simulink library "lib_orbittrance"  (Simulink 7.7)
settings: Solver=ode45  StartTime=0.0  StopTime=10.0  RelTol=1e-3
undefined symbols (not defined in the file): Earth, earth_radius, WGS84
libraries: aerolibutil x7, lib_util x4, vrlib x4, lib_orbittrance x4, lib_astrodynamics x3, aerolibtransform2 x2, lib_env x1
settings Model: Creator=miyata  LastModifiedBy=yamaurashusaku

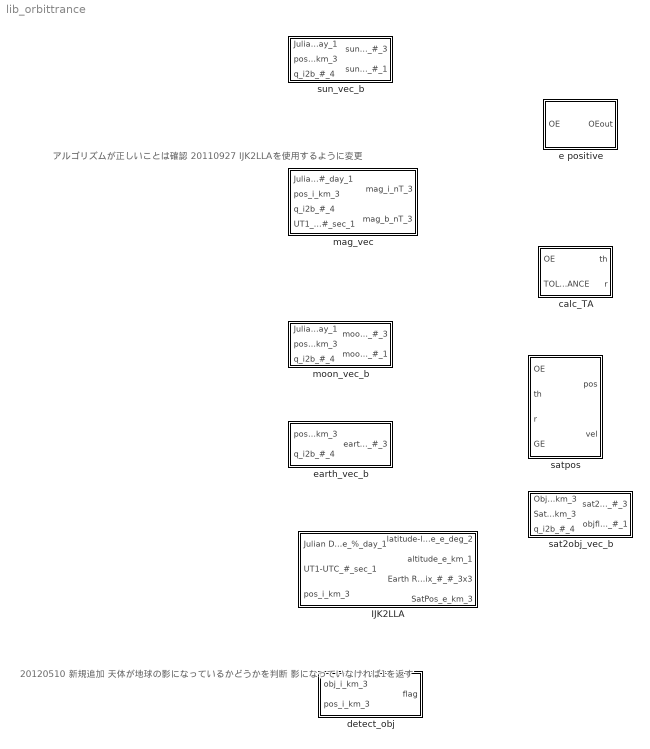
== system lib_orbittrance ==
  note: アルゴリズムが正しいことは確認
      | 20110927 IJK2LLAを使用するように変更
  note: 20120510 新規追加
      | 天体が地球の影になっているかどうかを判断
      | 影になっていなければ1を返す
  IJK2LLA : Subsystem
  calc_TA : Stateflow chart  TreatAsAtomicUnit=on
  detect_obj : Subsystem
  e positive : Stateflow chart  TreatAsAtomicUnit=on
  earth_vec_b : Subsystem
  mag_vec : Subsystem
  moon_vec_b : Subsystem
  sat2obj_vec_b : Subsystem
  satpos : Stateflow chart  TreatAsAtomicUnit=on
  sun_vec_b : Subsystem

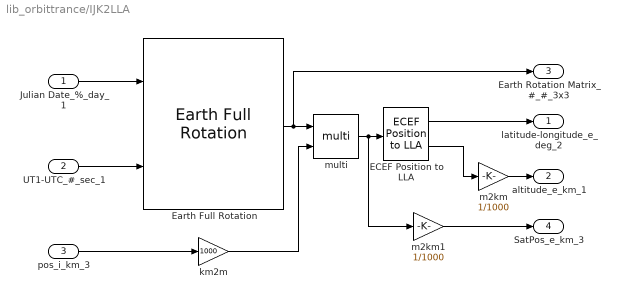
== system lib_orbittrance/IJK2LLA ==
  Julian Date_%_day_1 : Inport
  UT1-UTC_#_sec_1 : Inport  Port=2
  pos_i_km_3 : Inport  Port=3
  ECEF Position to LLA : aerolibtransform2/ECEF Position to LLA  units=Metric (MKS)  ptype=Earth (WGS84)  F=1/298.257223563  R=6378137
  Earth Full Rotation : lib_astrodynamics/Earth Full Rotation
  km2m : Gain  Gain=1000
  m2km : Gain  Gain=1/1000
  m2km1 : Gain  Gain=1/1000
  multi : lib_util/multi
  latitude-longitude_e_deg_2 : Outport
  altitude_e_km_1 : Outport  Port=2
  Earth Rotation Matrix_#_#_3x3 : Outport  Port=3
  SatPos_e_km_3 : Outport  Port=4
  wires:
  Julian Date_%_day_1/1 -> Earth Full Rotation/1
  UT1-UTC_#_sec_1/1 -> Earth Full Rotation/2
  pos_i_km_3/1 -> km2m/1
  Earth Full Rotation/1 -> multi/1, Earth Rotation Matrix_#_#_3x3/1
  km2m/1 -> multi/2
  multi/1 -> ECEF Position to LLA/1, m2km1/1
  ECEF Position to LLA/1 -> latitude-longitude_e_deg_2/1
  ECEF Position to LLA/2 -> m2km/1
  m2km/1 -> altitude_e_km_1/1
  m2km1/1 -> SatPos_e_km_3/1

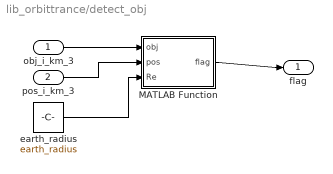
== system lib_orbittrance/detect_obj ==
  obj_i_km_3 : Inport
  pos_i_km_3 : Inport  Port=2
  MATLAB Function : Stateflow chart  TreatAsAtomicUnit=on
  earth_radius : Constant  Value=earth_radius
  flag : Outport
  wires:
  MATLAB Function/1(flag) -> flag/1
  obj_i_km_3/1 -> MATLAB Function/1(obj)
  pos_i_km_3/1 -> MATLAB Function/2(pos)
  earth_radius/1 -> MATLAB Function/3(Re)

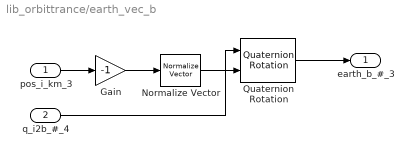
== system lib_orbittrance/earth_vec_b ==
  pos_i_km_3 : Inport
  q_i2b_#_4 : Inport  Port=2
  Gain : Gain  Gain=-1
  Normalize Vector : vrlib/Utilities/Normalize Vector  maxzero=0
  Quaternion Rotation : aerolibutil/Quaternion Rotation
  earth_b_#_3 : Outport
  wires:
  Normalize Vector/1 -> Quaternion Rotation/2
  Quaternion Rotation/1 -> earth_b_#_3/1
  q_i2b_#_4/1 -> Quaternion Rotation/1
  pos_i_km_3/1 -> Gain/1
  Gain/1 -> Normalize Vector/1

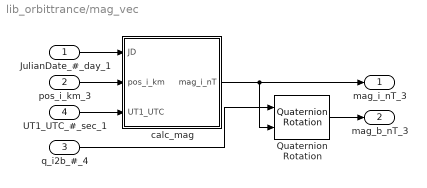
== system lib_orbittrance/mag_vec ==
  JulianDate_#_day_1 : Inport
  pos_i_km_3 : Inport  Port=2
  q_i2b_#_4 : Inport  Port=3
  UT1_UTC_#_sec_1 : Inport  Port=4
  Quaternion Rotation : aerolibutil/Quaternion Rotation  SystemSampleTime=-1
  calc_mag : Subsystem
  mag_i_nT_3 : Outport
  mag_b_nT_3 : Outport  Port=2
  wires:
  calc_mag/1(mag_i_nT) -> mag_i_nT_3/1, Quaternion Rotation/2
  JulianDate_#_day_1/1 -> calc_mag/1(JD)
  pos_i_km_3/1 -> calc_mag/2(pos_i_km)
  q_i2b_#_4/1 -> Quaternion Rotation/1
  Quaternion Rotation/1 -> mag_b_nT_3/1
  UT1_UTC_#_sec_1/1 -> calc_mag/3(UT1_UTC)

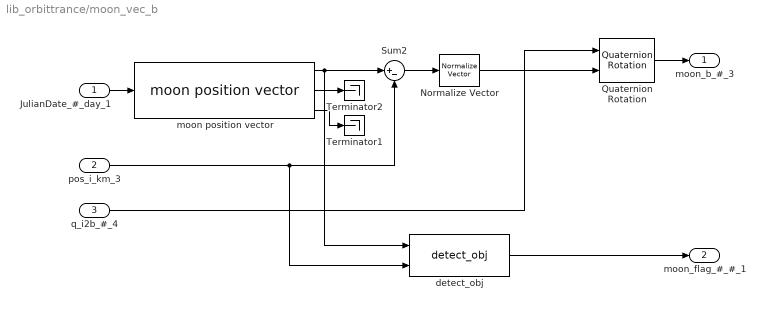
== system lib_orbittrance/moon_vec_b ==
  JulianDate_#_day_1 : Inport
  pos_i_km_3 : Inport  Port=2
  q_i2b_#_4 : Inport  Port=3
  Normalize Vector : vrlib/Utilities/Normalize Vector  maxzero=0
  Quaternion Rotation : aerolibutil/Quaternion Rotation
  Sum2 : Sum  Inputs=|+-
  Terminator1 : Terminator
  Terminator2 : Terminator
  detect_obj : lib_orbittrance/detect_obj
  moon position vector : lib_astrodynamics/moon position vector
  moon_b_#_3 : Outport
  moon_flag_#_#_1 : Outport  Port=2
  wires:
  moon position vector/2 -> Terminator2/1
  Normalize Vector/1 -> Quaternion Rotation/2
  moon position vector/1 -> Sum2/1, detect_obj/1
  Sum2/1 -> Normalize Vector/1
  Quaternion Rotation/1 -> moon_b_#_3/1
  JulianDate_#_day_1/1 -> moon position vector/1
  q_i2b_#_4/1 -> Quaternion Rotation/1
  moon position vector/3 -> Terminator1/1
  pos_i_km_3/1 -> Sum2/2, detect_obj/2
  detect_obj/1 -> moon_flag_#_#_1/1

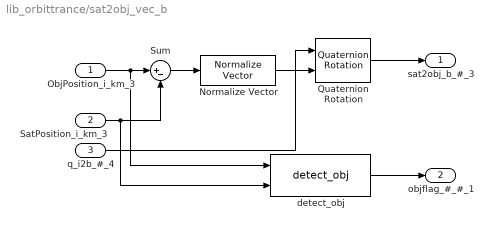
== system lib_orbittrance/sat2obj_vec_b ==
  ObjPosition_i_km_3 : Inport
  SatPosition_i_km_3 : Inport  Port=2
  q_i2b_#_4 : Inport  Port=3
  Normalize Vector : vrlib/Utilities/Normalize Vector  maxzero=0
  Quaternion Rotation : aerolibutil/Quaternion Rotation
  Sum : Sum  Inputs=|+-
  detect_obj : lib_orbittrance/detect_obj
  sat2obj_b_#_3 : Outport
  objflag_#_#_1 : Outport  Port=2
  wires:
  ObjPosition_i_km_3/1 -> Sum/1, detect_obj/1
  SatPosition_i_km_3/1 -> Sum/2, detect_obj/2
  Sum/1 -> Normalize Vector/1
  Normalize Vector/1 -> Quaternion Rotation/2
  q_i2b_#_4/1 -> Quaternion Rotation/1
  Quaternion Rotation/1 -> sat2obj_b_#_3/1
  detect_obj/1 -> objflag_#_#_1/1

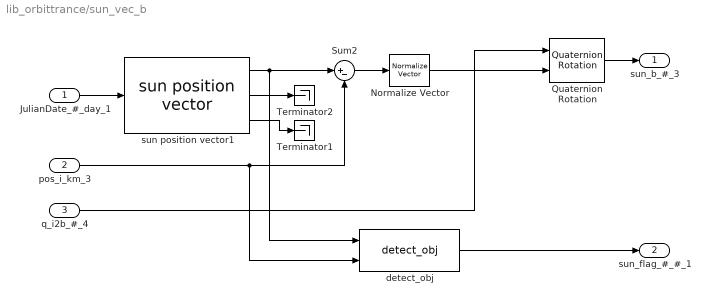
== system lib_orbittrance/sun_vec_b ==
  JulianDate_#_day_1 : Inport
  pos_i_km_3 : Inport  Port=2
  q_i2b_#_4 : Inport  Port=3
  Normalize Vector : vrlib/Utilities/Normalize Vector  maxzero=0
  Quaternion Rotation : aerolibutil/Quaternion Rotation
  Sum2 : Sum  Inputs=|+-
  Terminator1 : Terminator
  Terminator2 : Terminator
  detect_obj : lib_orbittrance/detect_obj
  sun position vector1 : lib_astrodynamics/sun position vector
  sun_b_#_3 : Outport
  sun_flag_#_#_1 : Outport  Port=2
  wires:
  sun position vector1/2 -> Terminator2/1
  Normalize Vector/1 -> Quaternion Rotation/2
  sun position vector1/1 -> Sum2/1, detect_obj/1
  Sum2/1 -> Normalize Vector/1
  Quaternion Rotation/1 -> sun_b_#_3/1
  JulianDate_#_day_1/1 -> sun position vector1/1
  q_i2b_#_4/1 -> Quaternion Rotation/1
  sun position vector1/3 -> Terminator1/1
  pos_i_km_3/1 -> Sum2/2, detect_obj/2
  detect_obj/1 -> sun_flag_#_#_1/1

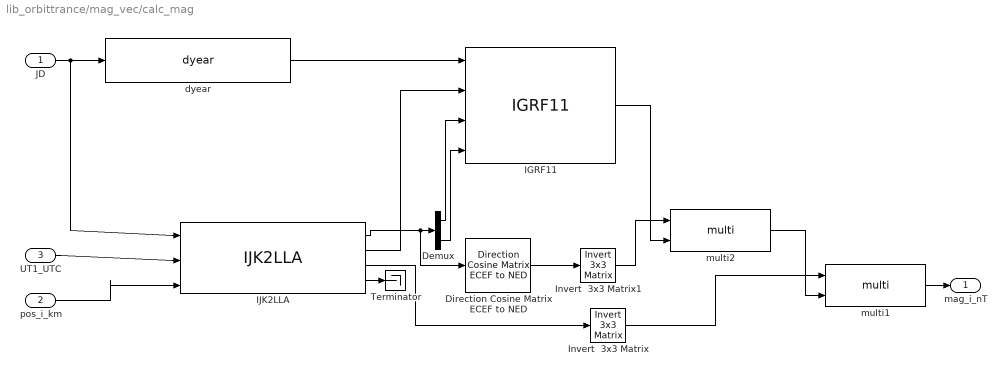
== system lib_orbittrance/mag_vec/calc_mag ==
  JD : Inport
  pos_i_km : Inport  Port=2
  UT1_UTC : Inport  Port=3
  Demux : Demux  Outputs=2
  Direction Cosine Matrix ECEF to NED : aerolibtransform2/Direction Cosine Matrix ECEF to NED
  IGRF11 : lib_env/IGRF11
  IJK2LLA : lib_orbittrance/IJK2LLA
  Invert  3x3 Matrix : aerolibutil/Invert  3x3 Matrix
  Invert  3x3 Matrix1 : aerolibutil/Invert  3x3 Matrix
  Terminator : Terminator
  dyear : lib_util/dyear
  multi1 : lib_util/multi
  multi2 : lib_util/multi
  mag_i_nT : Outport
  wires:
  JD/1 -> dyear/1, IJK2LLA/1
  dyear/1 -> IGRF11/1
  IJK2LLA/1 -> Demux/1, Direction Cosine Matrix ECEF to NED/1
  multi1/1 -> mag_i_nT/1
  Invert  3x3 Matrix/1 -> multi1/1
  UT1_UTC/1 -> IJK2LLA/2
  Direction Cosine Matrix ECEF to NED/1 -> Invert  3x3 Matrix1/1
  IJK2LLA/2 -> IGRF11/2
  Demux/1 -> IGRF11/3
  Demux/2 -> IGRF11/4
  Invert  3x3 Matrix1/1 -> multi2/1
  IGRF11/1 -> multi2/2
  multi2/1 -> multi1/2
  pos_i_km/1 -> IJK2LLA/3
  IJK2LLA/3 -> Invert  3x3 Matrix/1
  IJK2LLA/4 -> Terminator/1

== matlab function e positive ==
  data: OE input double; OEout output double
function OEout = fcn(OE)
%#codegen

a  = OE(1);         % semimajor axis [km]
e  = OE(2);         % eccentricity
i  = OE(3); % inclination [rad] -2*pi*floor(OE(1,4)/2/pi)
W  = OE(4); % - 2.0 * pi * floor(OE(4)/2.0/pi); % right ascension of the ascending node [rad] 
ww = OE(5); % - 2.0 * pi * floor(OE(5)/2.0/pi); % argument of perigee [rad] 
M  = OE(6); % - 2.0 * pi * floor(OE(6)/2.0/pi); % mean anomaly at epoch [rad]

if e < 0
    e = -e;
    ww = ww + pi;
    %ww = ww - 2.0 * pi * floor(ww/2.0/pi);
    M = M + pi;
    %M = M-2*pi*floor(M/2/pi);
end

W  = W - 2.0 * pi * floor(W/2.0/pi); % right ascension of the ascending node [rad]
ww = ww - 2.0 * pi * floor(ww/2.0/pi); % argument of perigee [rad] 
M  = M - 2.0 * pi * floor(M/2.0/pi); % mean anomaly at epoch [rad]

OEout=[a,e,i,W,ww,M];

== matlab function detect_obj/MATLAB Function ==
  data: obj input double; flag output double; pos input double; Re input double
function flag = detect_obj(obj,pos,Re)
%#codegen

obj = obj / norm(obj);
norm_pos = norm(pos);
proj_pos = pos' * obj;

flag = 0;

if proj_pos > 0 || norm_pos^2 - proj_pos^2 > Re^2
    flag = 1;
end

== matlab function calc_TA ==
  data: OE input double; th output double; TOLERANCE input double; r output double
function [th,r] = MOE_(OE,TOLERANCE)
%#codegen

a=OE(1);         % semimajor axis [km]
e=OE(2);         % eccentricity
i=OE(3); % inclination [rad] -2*pi*floor(OE(1,4)/2/pi)
W=OE(4); %-2*pi*floor(OE(4)/2/pi); % right ascension of the ascending node [rad] 
ww=OE(5); %-2*pi*floor(OE(5)/2/pi); % argument of perigee [rad] 
M=OE(6); %-2*pi*floor(OE(6)/2/pi); % mean anomaly at epoch [rad]

q = a * (1.0 - e);       % perigee distance [km]

%%%%%%%%%%%%%%%%%%%%%%%%%%%%%%%%%%%%%%%%%%%%%%%%%%%%%%%%%%%%%%%%%%%%%%%%%%%
%     calculate true anomaly th                                           %
%     calculate true distance r                                           %
%%%%%%%%%%%%%%%%%%%%%%%%%%%%%%%%%%%%%%%%%%%%%%%%%%%%%%%%%%%%%%%%%%%%%%%%%%%

if ( e == 0.0 )
    th = M;
    r = a;
elseif ( e == 1.0 )
    s = M;
    s2 = s * s;
    s3 = s2 * s;
    s = ( 2.0 * s3 + M ) / ( 3.0 * ( s2 + 1.0 ) );
    delta = s3 + 3.0 * s - M;
    while ( abs ( delta ) > TOLERANCE )
        s2 = s * s;
        s3 = s2 * s;
        s = ( 2.0 * s3 + M ) / ( 3.0 * ( s2 + 1.0 ) );
        delta = s3 + 3.0 * s - M;
    end
    th = 2.0 * atan ( s );
    r = q * ( 1.0 + s2 );
else
    %M = M-2*pi*floor(M/2/pi);
    ea = M;
    delta = ea - e * sin ( ea ) - M;
    while ( abs ( delta ) > TOLERANCE )
        ea = ea- delta / ( 1.0 - e * cos ( ea ) );
        delta = ea - e * sin ( ea ) - M;
    end
    th = 2.0 * atan ( sqrt ( ( 1.0 + e ) / ( 1.0 - e ) ) * tan ( ea / 2.0 ) );
    r = q * ( 1.0 + e ) / ( 1.0 + e * cos ( th ) );
end
  
th = th - 2.0 * pi * floor(th/2.0/pi);

== matlab function satpos ==
  data: OE input double; pos output double; th input double; r input double; GE input double; vel output double
function [pos,vel]  = sat_pos(OE,th,r,GE)
%#codegen
%calculate sat pos and vel

a = OE(1);
e = OE(2); 
W = OE(4);
i = OE(3);
ww = OE(5);

u = ww + th;
p = a * (1.0 -e * e);
h = sqrt(GE * p);

cu = cos(u);
su = sin(u);
ci = cos(i);
si = sin(i);
cW = cos(W);
sW = sin(W);

x = r * (cu * cW - su * ci * sW);
y = r * (cu * sW + su * ci * cW);
z = r * su * si;

pos = [x; y; z];

r_dot = h / a / (1.0 - e * e) * e * sin(th);
f_dot = h / r / r;
%   vx = r_dot*R(1,1)+r*f_dot*R(1,2); %/* vx[km/s] */
%   vy = r_dot*R(2,1)+r*f_dot*R(2,2); %/* vy[km/s] */
%   vz = r_dot*R(3,1)+r*f_dot*R(3,2); %/* vz[km/s] */
vx = r_dot * (cW * cu - sW * su * ci)+ r * f_dot * (-cW * su - sW * cu * ci); %/* vx[km/s] */
vy = r_dot * (sW * cu + cW * su * ci)+ r * f_dot * (-sW * su + cW * cu * ci); %/* vy[km/s] */
vz = r_dot * su * si + r * f_dot * cu * si; %/* vz[km/s] */
vel=[vx; vy; vz];
